simulink model "test_model"  (R2014a)
settings: Solver=ode45  StartTime=0.0  StopTime=10  RelTol=1e-3
model workspace: external: MATLAB File C:\Users\Iseberg-2\Documents\MATLAB\Model_01\Init_Model_01.m (data not in the file)
values from neighbouring files (symbols this model uses):
  p_x = (i_yy - i_zz)/i_xx    (= 0.75)    [Init_Model_01.m]    (also in Init_Model_02_Simulink.m)
  p_y = (i_zz - i_xx)/i_yy    (= 0.125)    [Init_Model_01.m]    (also in Init_Model_02_Simulink.m)
  p_z = (i_xx - i_yy)/i_zz    (= -0.8)    [Init_Model_01.m]    (also in Init_Model_02_Simulink.m)
  X_a_0 = [q_1_0;q_2_0;q_3_0;q_0_0;om_x_0;om_y_0;om_z_0;p_x_0;p_y_0;p_z_0;r_x_0;r_y_0;r_z_0;r_dot_x_0;r_dot_y_0;r_dot_z_0;rho;ita]    [Init_Model_01.m]    (also in Init_Model_02_Simulink.m = [q_1_0;q_2_0;q_3_0;q_0_0;om_x_0;om_y_0;om_z_0;r_x_0;r_y_0;r_)
settings Model: Creator=Iseberg-2  LastModifiedBy=Iseberg-2

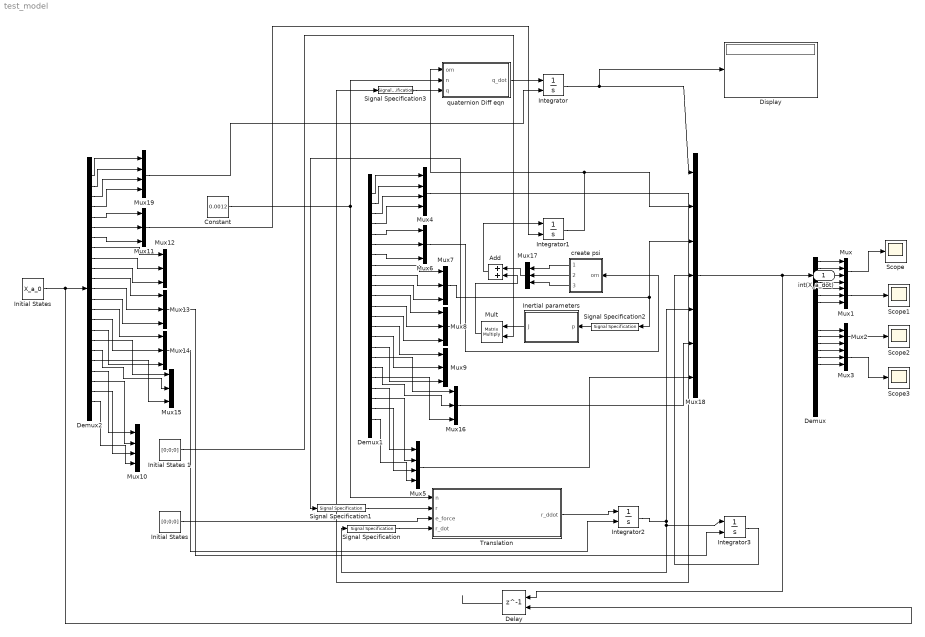
== system test_model ==
  Add : Sum
  Constant : Constant  Value=0.0012
  Delay : Delay  DelayLength=1  InitialConditionSource=Input port  InitialCondition=0
      settings: InputPortMap=u0,p4
  Demux : Demux  Outputs=23
  Demux1 : Demux  Outputs=23
  Demux2 : Demux  Outputs=23
  Display : Display
  Inertial parameters : MATLAB Function  TreatAsAtomicUnit=on
  Initial States : Constant  Value=[0;0;0]
  "Initial States " : Constant  Value=X_a_0
  Initial States 1 : Constant  Value=[0;0;0]
  Integrator{,1..3} (4 alike) : Integrator  InitialConditionSource=external
  Mult : Product  Inputs=**  Multiplication=Matrix(*)
  Mux{,4..5,10,19} (5 alike) : Mux
  Mux{1..3,6..9,11..17} (14 alike) : Mux  Inputs=3
  Mux18 : Mux  Inputs=7
  Scope{,1..3} (4 alike) : Scope
      Scope2 settings: SaveName=ScopeData2
      Scope3 settings: SaveName=ScopeData3
  Signal Specification : SignalSpecification  OutDataTypeStr=double  Dimensions=3
  Signal Specification1 : SignalSpecification  OutDataTypeStr=double  Dimensions=3
  Signal Specification2 : SignalSpecification  OutDataTypeStr=double  Dimensions=3
  Signal Specification3 : SignalSpecification  OutDataTypeStr=double  Dimensions=4
  Translation : MATLAB Function  TreatAsAtomicUnit=on
  create psi : Subsystem
  quaternion Diff eqn : MATLAB Function  TreatAsAtomicUnit=on
  int(X_a_dot) : Outport
  wires:
  Demux/1 -> Mux/1
  Demux/2 -> Mux/2
  Demux/3 -> Mux/3
  Demux/4 -> Mux/4
  Mux/1 -> Scope/1
  Demux/5 -> Mux1/1
  Demux/6 -> Mux1/2
  Demux/7 -> Mux1/3
  Mux1/1 -> Scope1/1
  Demux/11 -> Mux2/1
  Demux/12 -> Mux2/2
  Demux/13 -> Mux2/3
  Mux2/1 -> Scope2/1
  Demux/14 -> Mux3/1
  Demux/15 -> Mux3/2
  Demux/16 -> Mux3/3
  Mux3/1 -> Scope3/1
  Demux1/1 -> Mux4/1
  Demux1/2 -> Mux4/2
  Demux1/3 -> Mux4/3
  Demux1/4 -> Mux4/4
  Demux1/20 -> Mux5/1
  Demux1/21 -> Mux5/2
  Demux1/22 -> Mux5/3
  Demux1/23 -> Mux5/4
  Demux1/5 -> Mux6/1
  Demux1/6 -> Mux6/2
  Demux1/7 -> Mux6/3
  Demux1/8 -> Mux7/1
  Demux1/9 -> Mux7/2
  Demux1/10 -> Mux7/3
  Demux1/11 -> Mux8/1
  Demux1/12 -> Mux8/2
  Demux1/13 -> Mux8/3
  Demux1/14 -> Mux9/1
  Demux1/15 -> Mux9/2
  Demux1/16 -> Mux9/3
  Demux1/17 -> Mux16/1
  Demux1/18 -> Mux16/2
  Demux1/19 -> Mux16/3
  Integrator/1 -> Display/1, Mux18/1
  Integrator1/1 -> Mux18/2, quaternion Diff eqn/1(om)
  Mult/1 -> Add/2
  create psi/1(psi_1) -> Mux17/1
  create psi/2(psi_2) -> Mux17/2
  create psi/3("psi_3 ") -> Mux17/3
  Mux17/1 -> Add/1
  Add/1 -> Integrator1/1
  Translation/1(r_ddot) -> Integrator2/1
  Initial States/1 -> Translation/3(e_force)
  Integrator3/1 -> Mux18/4
  Mux16/1 -> Mux18/6
  Mux5/1 -> Mux18/7
  Inertial parameters/1(J) -> Mult/1
  Constant/1 -> Translation/1(n), quaternion Diff eqn/2(n)
  Mux18/1 -> Delay/1, int(X_a_dot)/1
  Mux7/1 -> Mux18/3, Signal Specification2/1
  Initial States 1/1 -> Mult/2
  Signal Specification/1 -> Translation/4(r_dot)
  Signal Specification1/1 -> Translation/2(r)
  Signal Specification2/1 -> Inertial parameters/1(p)
  Signal Specification3/1 -> quaternion Diff eqn/3(q)
  quaternion Diff eqn/1(q_dot) -> Integrator/1
  Integrator2/1 -> Integrator3/1, Signal Specification/1, Mux18/5
  Demux2/1 -> Mux19/1
  Demux2/2 -> Mux19/2
  Demux2/3 -> Mux19/3
  Demux2/4 -> Mux19/4
  Demux2/20 -> Mux10/1
  Demux2/21 -> Mux10/2
  Demux2/22 -> Mux10/3
  Demux2/23 -> Mux10/4
  Demux2/5 -> Mux11/1
  Demux2/6 -> Mux11/2
  Demux2/7 -> Mux11/3
  Demux2/8 -> Mux12/1
  Demux2/9 -> Mux12/2
  Demux2/10 -> Mux12/3
  Demux2/11 -> Mux13/1
  Demux2/12 -> Mux13/2
  Demux2/13 -> Mux13/3
  Demux2/14 -> Mux14/1
  Demux2/15 -> Mux14/2
  Demux2/16 -> Mux14/3
  Demux2/17 -> Mux15/1
  Demux2/18 -> Mux15/2
  Demux2/19 -> Mux15/3
  "Initial States "/1 -> Delay/2, Demux2/1
  Mux19/1 -> Integrator/2
  Mux11/1 -> Integrator1/2
  Mux4/1 -> Signal Specification3/1
  Mux6/1 -> create psi/1(om)
  Mux13/1 -> Integrator3/2
  Mux14/1 -> Integrator2/2
  Mux8/1 -> Signal Specification1/1
  ? -> Demux1/1
  Delay/1 -> ?

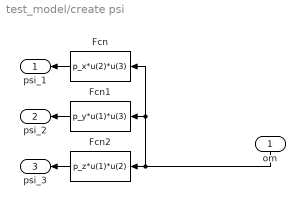
== system test_model/create psi ==
  om : Inport
  Fcn : Fcn  Expr=p_x*u(2)*u(3)
  Fcn1 : Fcn  Expr=p_y*u(1)*u(3)
  Fcn2 : Fcn  Expr=p_z*u(1)*u(2)
  psi_1 : Outport
  psi_2 : Outport  Port=2
  "psi_3 " : Outport  Port=3
  wires:
  Fcn/1 -> psi_1/1
  Fcn2/1 -> "psi_3 "/1
  om/1 -> Fcn/1, Fcn1/1, Fcn2/1
  Fcn1/1 -> psi_2/1

== matlab function test_model/quaternion Diff eqn ==
  data: om input; q_dot output; n input; q input
function q_dot  = fn_Create_qdot(om, n, q)
    v_n = [0;0;n];
    q_n = [v_n;0];
    q_om = [om;0];
    Tensor_om = fn_CrossTensor(q_om,0);
    Tensor_n = fn_CrossTensor(q_n,1);
    q_dot = (1/2)*(Tensor_om - Tensor_n)*q;
end

== matlab function test_model/Translation ==
  data: n input; r_ddot output; r input; e_force input; r_dot input
function r_ddot = fn_Compute_r_ddot(n,r,e_force,r_dot)
%#codegen
    parameter_gravitation = 398.6005e12;
    re = [(parameter_gravitation/n^2)^(1/3);0;0];
    v_n = [0;0;n];
    Tensor_n = fn_VectorToSkewSymmetricTensor(v_n);
    Term_1 = -2*Tensor_n*r_dot;
    Term_2 = Tensor_n*(Tensor_n*r);
    Term_3 = parameter_gravitation*(re + r)/(norm(re+r))^3;
    Term_4 = (n^2)*re;
    
    r_ddot = Term_1 - Term_2 - Term_3 + Term_4 + e_force;
end

== matlab function test_model/Inertial parameters ==
  data: p input; J output
function J = fn_Create_J(p)
%#codegen
    J = [1,0,0;0, (1-p(2))/(1+p(1)), 0;0, 0, (1+p(3))/(1-p(1))];
end
